simulink model "prochazkaModel"  (R2022b)
settings: Solver=VariableStepAuto  StartTime=0.0  StopTime=10.0  MaxStep=0.2  RelTol=1e-3
settings Model: SimulationMode=accelerator  Creator=migpa  LastModifiedBy=migpa
settings SolverCC: AlgebraicLoopSolver=TrustRegion
settings DebuggingCC: UnconnectedInputMsg=warning  UnconnectedOutputMsg=warning  UnconnectedLineMsg=warning  SFMachineParentedDataDiag=warning
settings ModelReferenceCC: EnableRefExpFcnMdlSchedulingChecks=on
settings RTWCC: DLArmComputeVersion=19.05

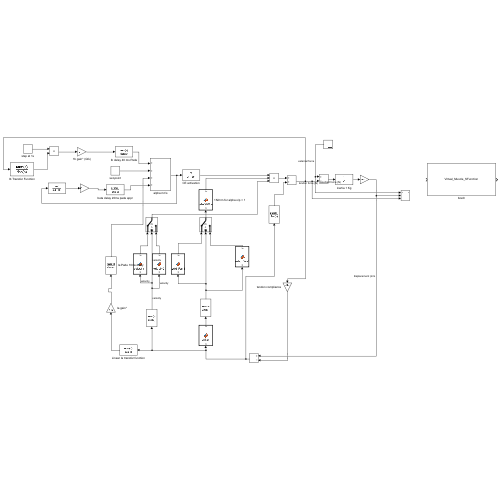
[thumbnail: Simulink's stored preview of the top-level diagram]
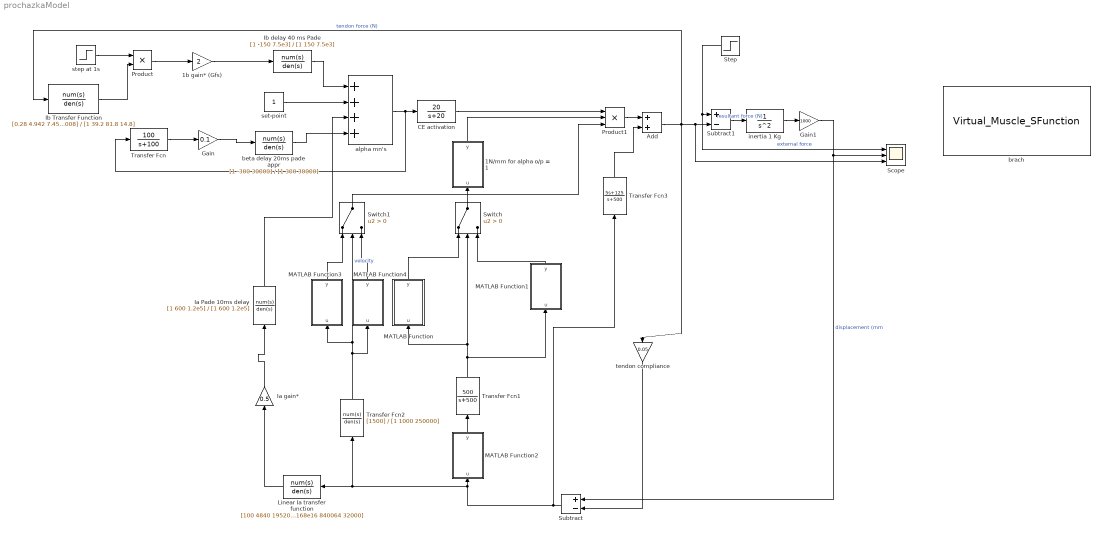
== system prochazkaModel ==
  1N/mm for alpha o/p = 1 : MATLAB Function  TreatAsAtomicUnit=on
  1b gain* (Gfs) : Gain  Gain=2
  Add : Sum
  CE activation : TransferFcn  Numerator=[20]  Denominator=[1 20]
  Gain : Gain  Gain=0.1
  Gain1 : Gain  Gain=1000
  Ia Pade 10ms delay : TransferFcn  Numerator=[1 600 1.2e5]  Denominator=[1 600 1.2e5]
  Ia gain* : Gain  Gain=0.5
  Ib Transfer Function : TransferFcn  Numerator=[0.28 4.942 7.455 1.008]  Denominator=[1 39.2 81.8 14.8]
  Ib delay 40 ms Pade : TransferFcn  Numerator=[1 -150 7.5e3]  Denominator=[1 150 7.5e3]
  Linear Ia transfer function : TransferFcn  Numerator=[100 4840 19520 7040]  Denominator=[1 2000.84 1.00168e16 840064 32000]
  MATLAB Function : MATLAB Function  TreatAsAtomicUnit=on
  MATLAB Function1 : MATLAB Function  TreatAsAtomicUnit=on
  MATLAB Function2 : MATLAB Function  TreatAsAtomicUnit=on
  MATLAB Function3 : MATLAB Function  TreatAsAtomicUnit=on
  MATLAB Function4 : MATLAB Function  TreatAsAtomicUnit=on
  Product : Product
  Product1 : Product  Inputs=3
  Scope : Scope  NumInputPorts=3
  Step : Step  Before=30  After=0  SampleTime=0
  Subtract : Sum  Inputs=+-
  Subtract1 : Sum  Inputs=+-
  Switch : Switch  Criteria=u2 > Threshold  SaturateOnIntegerOverflow=off  InputSameDT=off
  Switch1 : Switch  Criteria=u2 > Threshold  SaturateOnIntegerOverflow=off  InputSameDT=off
  Transfer Fcn : TransferFcn  Numerator=[100]  Denominator=[1 100]
  Transfer Fcn1 : TransferFcn  Numerator=[500]  Denominator=[1 500]
  Transfer Fcn2 : TransferFcn  Numerator=[1500]  Denominator=[1 1000 250000]
  Transfer Fcn3 : TransferFcn  Numerator=[5 125]  Denominator=[1 500]
  alpha mn's : Sum  Inputs=++++
  beta delay 20ms pade appr : TransferFcn  Numerator=[1 -300 30000]  Denominator=[1 300 30000]
  brach : S-Function  FunctionName=Virtual_Muscle_SFunction  Parameters=TOFMUSFIB SARCLEN SPTEN VISC C1 K1 LR1 C2 K2 LR2 CT KT LRT RRANK V05 F05 FMIN FMAX FLOMEGA FLBETA FLRHO VMAX CV0 CV1 AV0 AV1 AV2 BV AF NF0 NF1 TL TF1 TF2 TF3 TF4 AS1 AS2 TS CY VY TY CH0 CH1 CH2 CH3 RTYPE ADDPORTS MMASS FASCL0 TENDL0T LPATH UR NUMOFUNITS FPCSA UPCSA APPORTMTD GEOPCSA  SFunctionDeploymentMode=off  EnableBusSupport=off  mask(Virtual Muscle Parameters){RTYPE=3, ADDPORTS=[1  0  0  0  0], FASCL0=13, TENDL0T=4, LPATH=18, MMASS=10, UR=0.8, SPTEN=31.8, VISC=0.01, SARCLEN=2.7, C1=23, K1=0.046, LR1=1.17, C2=-0.02, K2=-21.0375, LR2=0.70222, CT=27.8, KT=0.0047, LRT=0.964, TOFMUSFIB=0, FPCSA=[], NUMOFUNITS=[], APPORTMTD=3, GEOPCSA=0, UPCSA=[], RRANK=[], V05=[], F05=[], FMIN=[], FMAX=[], FLOMEGA=[], FLBETA=[], FLRHO=[], VMAX=[], CV0=[], CV1=[], AV0=[], AV1=[], AV2=[], BV=[], AF=[], NF0=[], NF1=[], TL=[], TF1=[], TF2=[], TF3=[], TF4=[], AS1=[], AS2=[], TS=[], CY=[], VY=[], TY=[], CH0=[], CH1=[], CH2=[], CH3=[]}
      mask prompts: RTYPE "Recruitment Type (2-Natural Discrete, 3-Natural Continuous, 4-Intramuscular FES)"; ADDPORTS "Additional Outputs"; FASCL0 "Optimal Fascicle Length (cm)"; TENDL0T "Optimal Tendon Length (cm)"; LPATH "Maximum Path Length (cm)"; MMASS "Muscle Mass (g)"; UR "Maximum Recruitment Activation (Ur)"; SPTEN "Specific Tension (N/cm2)"; VISC "Viscosity (part of FPE1)"; SARCLEN "Optimal sarcomere length (um)"; C1 "C1 (FPE1)"; K1 "K1 (FPE1)"; LR1 "LR1 (FPE1)"; C2 "C2 (FPE2)"; K2 "K2 (FPE2)"; LR2 "LR2 (FPE2)"; CT "CT (FSE)"; KT "KT (FSE)"; LRT "LRT (FSE)"; TOFMUSFIB "Number of Fiber Types"; FPCSA "Fractional PCSA for Each Muscle Fiber Type"; NUMOFUNITS "Number of motor units in each muscle fiber type"; APPORTMTD "Apportion Method (1-Manual, 2-Default, 3-Geometric, 4-Equal)"; GEOPCSA "Fractional increase in PCSA for Geometric Apportion Method"; UPCSA "PCSA for Each Motor Unit (Manual changes effective only for Apportion Method 1"; RRANK "Recruitment Rank"; V05 "V0.5 (L0/s)"; F05 "f0.5 (pps)"; FMIN "fmin (f0.5)"; FMAX "fmax (f0.5)"; FLOMEGA "FL_omega"; FLBETA "FL_beta"; FLRHO "FL_rho"
  inertia 1 Kg : TransferFcn  Denominator=[1 0 0]
  set-point : Constant
  step at 1s : Step  SampleTime=0
  tendon compliance : Gain  Gain=0.05
  wires:
  Transfer Fcn/1 -> Gain/1
  step at 1s/1 -> Product/1
  Ib Transfer Function/1 -> Product/2
  set-point/1 -> alpha mn's/2
  Product/1 -> 1b gain* (Gfs)/1
  1b gain* (Gfs)/1 -> Ib delay 40 ms Pade/1
  Gain/1 -> beta delay 20ms pade appr/1
  alpha mn's/1 -> Transfer Fcn/1, CE activation/1
  Switch/1 -> 1N/mm for alpha o/p = 1/1(u)
  CE activation/1 -> Product1/1
  MATLAB Function/1(y) -> Switch/1
  MATLAB Function1/1(y) -> Switch/3
  Transfer Fcn1/1 -> MATLAB Function1/1(u), MATLAB Function/1(u), Switch/2
  MATLAB Function2/1(y) -> Transfer Fcn1/1
  Subtract/1 -> Transfer Fcn2/1, Linear Ia transfer function/1, MATLAB Function2/1(u), Transfer Fcn3/1
  tendon compliance/1 -> Subtract/2
  Ia gain*/1 -> Ia Pade 10ms delay/1
  Linear Ia transfer function/1 -> Ia gain*/1
  Ia Pade 10ms delay/1 -> alpha mn's/3
  1N/mm for alpha o/p = 1/1(y) -> Product1/2
  Transfer Fcn2/1 -> MATLAB Function4/1(u), MATLAB Function3/1(u), Switch1/2  "velocity"
  MATLAB Function3/1(y) -> Switch1/1
  MATLAB Function4/1(y) -> Switch1/3
  Switch1/1 -> Product1/3
  Product1/1 -> Add/1
  Transfer Fcn3/1 -> Add/2
  Add/1 -> tendon compliance/1, Ib Transfer Function/1, Scope/3, Subtract1/2  "tendon force (N)"
  Subtract1/1 -> inertia 1 Kg/1  "resultant force (N)"
  inertia 1 Kg/1 -> Gain1/1
  Gain1/1 -> Subtract/1, Scope/2  "displacement (mm"
  Step/1 -> Scope/1, Subtract1/1  "external force"
  Ib delay 40 ms Pade/1 -> alpha mn's/1
  beta delay 20ms pade appr/1 -> alpha mn's/4

== matlab function prochazkaModel/MATLAB Function ==
  data: u input; y output
function y = switchFun1(u)

y = 1-exp(-0.15*u);

== matlab function prochazkaModel/MATLAB Function2 ==
  data: u input; y output
function y = offset(u)

y = u-8;

== matlab function prochazkaModel/1N//mm for alpha o//p = 1 ==
  data: u input; y output
function y = parallelStiffness(u)

y = (10*u)+7;

== matlab function prochazkaModel/MATLAB Function3 ==
  data: u input; y output
function y = velocity1(u)

y = 1+(0.5*(1-exp(-1.5*u)));

== matlab function prochazkaModel/MATLAB Function4 ==
  data: u input; y output
function y = velocity2(u)

y = 1/(1-u);

== matlab function prochazkaModel/MATLAB Function1 ==
  data: u input; y output
function y = switchFun2(u)

y = -1+exp(0.15*u);
